simulink model "obstacle_detection"  (R2022b)
settings: Solver=VariableStepAuto  StartTime=0.0  StopTime=10.0  RelTol=1e-3
values from neighbouring files (symbols this model uses):
  m = 12    [mpc.m]    (also in mpc_soln.m; qp_soln.m)
  N = 50    [mpc.m]    (also in mpc_caller.m = 20; qp_caller.m = params.N)
  X = [p; reshape(R, [9 1]); v; R'*w]    [mpc_caller.m]    (also in qp_caller.m)
undefined symbols (not defined in the file or in its folder): Y, Z
libraries: sm_lib x269, nesl_utility x117, simulink x2
(part 5 of 5)

== system obstacle_detection/q_dot ==
  RR_calf : Inport
  RL_calf : Inport  Port=2
  FR_calf : Inport  Port=3
  FL_calf : Inport  Port=4
  RR_thigh : Inport  Port=5
  RL_thigh : Inport  Port=6
  FR_thigh : Inport  Port=7
  FL_thigh : Inport  Port=8
  RR_hip : Inport  Port=9
  RL_hip : Inport  Port=10
  FR_hip : Inport  Port=11
  FL_hip : Inport  Port=12
  Scope : Scope  NumInputPorts=12
  Vector Concatenate : Concatenate  NumInputs=12
  joint vector : Outport
  wires:
  Vector Concatenate/1 -> joint vector/1
  FR_thigh/1 -> Scope/7, Vector Concatenate/7
  FL_hip/1 -> Scope/12, Vector Concatenate/12
  FL_calf/1 -> Scope/4, Vector Concatenate/4
  FL_thigh/1 -> Scope/8, Vector Concatenate/8
  FR_hip/1 -> Scope/11, Vector Concatenate/11
  RR_calf/1 -> Scope/1, Vector Concatenate/1
  RL_hip/1 -> Scope/10, Vector Concatenate/10
  FR_calf/1 -> Scope/3, Vector Concatenate/3
  RR_thigh/1 -> Scope/5, Vector Concatenate/5
  RL_calf/1 -> Scope/2, Vector Concatenate/2
  RL_thigh/1 -> Scope/6, Vector Concatenate/6
  RR_hip/1 -> Scope/9, Vector Concatenate/9

== system obstacle_detection/qd ==
  RR_calf : Inport
  RL_calf : Inport  Port=2
  FR_calf : Inport  Port=3
  FL_calf : Inport  Port=4
  RR_thigh : Inport  Port=5
  RL_thigh : Inport  Port=6
  FR_thigh : Inport  Port=7
  FL_thigh : Inport  Port=8
  RR_hip : Inport  Port=9
  RL_hip : Inport  Port=10
  FR_hip : Inport  Port=11
  FL_hip : Inport  Port=12
  Vector Concatenate : Concatenate  NumInputs=12
  Joint vector : Outport
  wires:
  Vector Concatenate/1 -> Joint vector/1
  FR_hip/1 -> Vector Concatenate/11
  RL_calf/1 -> Vector Concatenate/2
  FL_calf/1 -> Vector Concatenate/4
  RL_thigh/1 -> Vector Concatenate/6
  FL_thigh/1 -> Vector Concatenate/8
  RR_calf/1 -> Vector Concatenate/1
  RR_hip/1 -> Vector Concatenate/9
  FR_calf/1 -> Vector Concatenate/3
  RR_thigh/1 -> Vector Concatenate/5
  FL_hip/1 -> Vector Concatenate/12
  RL_hip/1 -> Vector Concatenate/10
  FR_thigh/1 -> Vector Concatenate/7

== system obstacle_detection/tau ==
  RR_calf : Inport
  RL_calf : Inport  Port=2
  FR_calf : Inport  Port=3
  FL_calf : Inport  Port=4
  RR_thigh : Inport  Port=5
  RL_thigh : Inport  Port=6
  FR_thigh : Inport  Port=7
  FL_thigh : Inport  Port=8
  RR_hip : Inport  Port=9
  RL_hip : Inport  Port=10
  FR_hip : Inport  Port=11
  FL_hip : Inport  Port=12
  Joint Torques : Scope  NumInputPorts=12
  Vector Concatenate : Concatenate  NumInputs=12
  joint vector : Outport
  wires:
  Vector Concatenate/1 -> joint vector/1
  FR_thigh/1 -> Joint Torques/7, Vector Concatenate/7
  FL_hip/1 -> Joint Torques/12, Vector Concatenate/12
  FL_calf/1 -> Joint Torques/4, Vector Concatenate/4
  FL_thigh/1 -> Joint Torques/8, Vector Concatenate/8
  FR_hip/1 -> Joint Torques/11, Vector Concatenate/11
  RR_calf/1 -> Joint Torques/1, Vector Concatenate/1
  RL_hip/1 -> Joint Torques/10, Vector Concatenate/10
  FR_calf/1 -> Joint Torques/3, Vector Concatenate/3
  RR_thigh/1 -> Joint Torques/5, Vector Concatenate/5
  RL_calf/1 -> Joint Torques/2, Vector Concatenate/2
  RL_thigh/1 -> Joint Torques/6, Vector Concatenate/6
  RR_hip/1 -> Joint Torques/9, Vector Concatenate/9

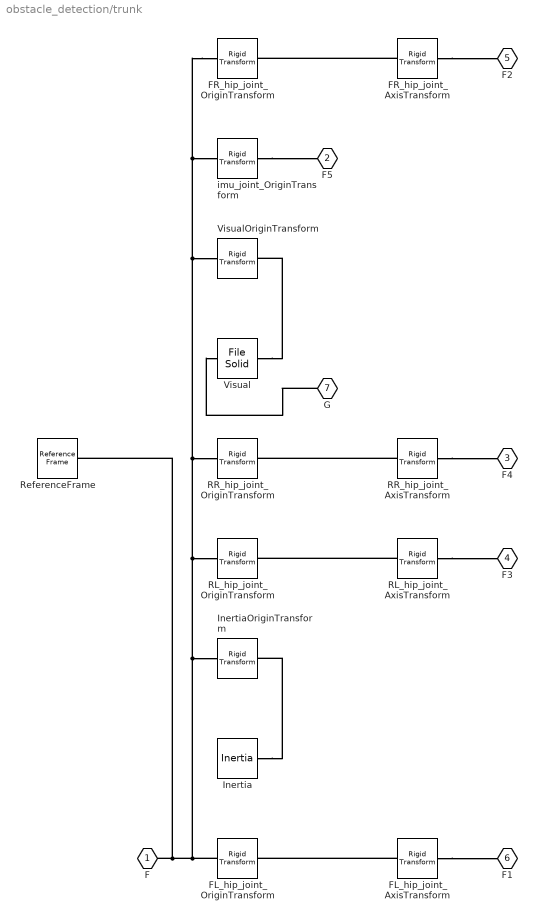
== system obstacle_detection/trunk ==
  FL_hip_joint_AxisTransform : sm_lib/Frames and Transforms/Rigid Transform  TranslationMethod=Cartesian  TranslationStandardOffset=0  TranslationLengthUnit=m  TranslationStandardAxis=+Z  TranslationCartesianOffset=[0, 0, 0]  TranslationROffset=0  TranslationROffsetUnits=m  TranslationZOffset=0  TranslationZOffsetUnits=m  TranslationThetaOffset=0  TranslationThetaOffsetUnits=deg  RotationMethod=ArbitraryAxis  RotationAngleUnits=rad  RotationStandardAxis=+Z  RotationAngle=1.570796326794897  RotationArbitraryAxis=[-0, 1, 0]  FollAlignAxisA=+X  BaseAlignAxisA=+Y  FollAlignAxisB=+Y  BaseAlignAxisB=+Z  RotationSequenceAxes=FollowerAxes  RotationSequence=XYX  RotationSequenceAngles=[0 0 0]  RotationSequenceAnglesUnits=deg  RotationMatrix=[1 0 0; 0 1 0; 0 0 1]  Quaternion=[1 0 0 0]
  FL_hip_joint_OriginTransform : sm_lib/Frames and Transforms/Rigid Transform  TranslationMethod=Cartesian  TranslationStandardOffset=0  TranslationLengthUnit=m  TranslationStandardAxis=+Z  TranslationCartesianOffset=[0.1805, 0.047, 0]  TranslationROffset=0  TranslationROffsetUnits=m  TranslationZOffset=0  TranslationZOffsetUnits=m  TranslationThetaOffset=0  TranslationThetaOffsetUnits=deg  RotationMethod=RotationSequence  RotationAngleUnits=deg  RotationStandardAxis=+Z  RotationAngle=0.0  RotationArbitraryAxis=[0 0 1]  FollAlignAxisA=+X  BaseAlignAxisA=+Y  FollAlignAxisB=+Y  BaseAlignAxisB=+Z  RotationSequenceAxes=BaseAxes  RotationSequence=XYZ  RotationSequenceAngles=[0, 0, 0]  RotationSequenceAnglesUnits=rad  RotationMatrix=[1 0 0; 0 1 0; 0 0 1]  Quaternion=[1 0 0 0]
  FR_hip_joint_AxisTransform : sm_lib/Frames and Transforms/Rigid Transform  TranslationMethod=Cartesian  TranslationStandardOffset=0  TranslationLengthUnit=m  TranslationStandardAxis=+Z  TranslationCartesianOffset=[0, 0, 0]  TranslationROffset=0  TranslationROffsetUnits=m  TranslationZOffset=0  TranslationZOffsetUnits=m  TranslationThetaOffset=0  TranslationThetaOffsetUnits=deg  RotationMethod=ArbitraryAxis  RotationAngleUnits=rad  RotationStandardAxis=+Z  RotationAngle=1.570796326794897  RotationArbitraryAxis=[-0, 1, 0]  FollAlignAxisA=+X  BaseAlignAxisA=+Y  FollAlignAxisB=+Y  BaseAlignAxisB=+Z  RotationSequenceAxes=FollowerAxes  RotationSequence=XYX  RotationSequenceAngles=[0 0 0]  RotationSequenceAnglesUnits=deg  RotationMatrix=[1 0 0; 0 1 0; 0 0 1]  Quaternion=[1 0 0 0]
  FR_hip_joint_OriginTransform : sm_lib/Frames and Transforms/Rigid Transform  TranslationMethod=Cartesian  TranslationStandardOffset=0  TranslationLengthUnit=m  TranslationStandardAxis=+Z  TranslationCartesianOffset=[0.1805, -0.047, 0]  TranslationROffset=0  TranslationROffsetUnits=m  TranslationZOffset=0  TranslationZOffsetUnits=m  TranslationThetaOffset=0  TranslationThetaOffsetUnits=deg  RotationMethod=RotationSequence  RotationAngleUnits=deg  RotationStandardAxis=+Z  RotationAngle=0.0  RotationArbitraryAxis=[0 0 1]  FollAlignAxisA=+X  BaseAlignAxisA=+Y  FollAlignAxisB=+Y  BaseAlignAxisB=+Z  RotationSequenceAxes=BaseAxes  RotationSequence=XYZ  RotationSequenceAngles=[0, 0, 0]  RotationSequenceAnglesUnits=rad  RotationMatrix=[1 0 0; 0 1 0; 0 0 1]  Quaternion=[1 0 0 0]
  Inertia : sm_lib/Body Elements/Inertia  InertiaType=Custom  Mass=6  MassUnits=kg  CenterOfMass=[0, 0, 0]  CenterOfMassUnits=m  MomentsOfInertia=[0.0158533, 0.0377999, 0.0456542]  MomentsOfInertiaUnits=kg*m^2  ProductsOfInertia=[-2.75e-05, -6.109999999999999e-05, -3.66e-05]  ProductsOfInertiaUnits=kg*m^2  GraphicType=None  MarkerShape=Inertia  MarkerSize=20  GraphicVisPropType=SimpleVisualProperties  GraphicDiffuseColor=[0.5 0.5 0.5]  GraphicSpecularColor=[0.5 0.5 0.5 1.0]  GraphicAmbientColor=[0.15 0.15 0.15 1.0]  GraphicEmissiveColor=[0.0 0.0 0.0 1.0]  GraphicShininess=75  GraphicOpacity=1.0
  InertiaOriginTransform : sm_lib/Frames and Transforms/Rigid Transform  TranslationMethod=Cartesian  TranslationStandardOffset=0  TranslationLengthUnit=m  TranslationStandardAxis=+Z  TranslationCartesianOffset=[0, 0.0041, -0.0005]  TranslationROffset=0  TranslationROffsetUnits=m  TranslationZOffset=0  TranslationZOffsetUnits=m  TranslationThetaOffset=0  TranslationThetaOffsetUnits=deg  RotationMethod=RotationSequence  RotationAngleUnits=deg  RotationStandardAxis=+Z  RotationAngle=0.0  RotationArbitraryAxis=[0 0 1]  FollAlignAxisA=+X  BaseAlignAxisA=+Y  FollAlignAxisB=+Y  BaseAlignAxisB=+Z  RotationSequenceAxes=BaseAxes  RotationSequence=XYZ  RotationSequenceAngles=[0, 0, 0]  RotationSequenceAnglesUnits=rad  RotationMatrix=[1 0 0; 0 1 0; 0 0 1]  Quaternion=[1 0 0 0]
  RL_hip_joint_AxisTransform : sm_lib/Frames and Transforms/Rigid Transform  TranslationMethod=Cartesian  TranslationStandardOffset=0  TranslationLengthUnit=m  TranslationStandardAxis=+Z  TranslationCartesianOffset=[0, 0, 0]  TranslationROffset=0  TranslationROffsetUnits=m  TranslationZOffset=0  TranslationZOffsetUnits=m  TranslationThetaOffset=0  TranslationThetaOffsetUnits=deg  RotationMethod=ArbitraryAxis  RotationAngleUnits=rad  RotationStandardAxis=+Z  RotationAngle=1.570796326794897  RotationArbitraryAxis=[-0, 1, 0]  FollAlignAxisA=+X  BaseAlignAxisA=+Y  FollAlignAxisB=+Y  BaseAlignAxisB=+Z  RotationSequenceAxes=FollowerAxes  RotationSequence=XYX  RotationSequenceAngles=[0 0 0]  RotationSequenceAnglesUnits=deg  RotationMatrix=[1 0 0; 0 1 0; 0 0 1]  Quaternion=[1 0 0 0]
  RL_hip_joint_OriginTransform : sm_lib/Frames and Transforms/Rigid Transform  TranslationMethod=Cartesian  TranslationStandardOffset=0  TranslationLengthUnit=m  TranslationStandardAxis=+Z  TranslationCartesianOffset=[-0.1805, 0.047, 0]  TranslationROffset=0  TranslationROffsetUnits=m  TranslationZOffset=0  TranslationZOffsetUnits=m  TranslationThetaOffset=0  TranslationThetaOffsetUnits=deg  RotationMethod=RotationSequence  RotationAngleUnits=deg  RotationStandardAxis=+Z  RotationAngle=0.0  RotationArbitraryAxis=[0 0 1]  FollAlignAxisA=+X  BaseAlignAxisA=+Y  FollAlignAxisB=+Y  BaseAlignAxisB=+Z  RotationSequenceAxes=BaseAxes  RotationSequence=XYZ  RotationSequenceAngles=[0, 0, 0]  RotationSequenceAnglesUnits=rad  RotationMatrix=[1 0 0; 0 1 0; 0 0 1]  Quaternion=[1 0 0 0]
  RR_hip_joint_AxisTransform : sm_lib/Frames and Transforms/Rigid Transform  TranslationMethod=Cartesian  TranslationStandardOffset=0  TranslationLengthUnit=m  TranslationStandardAxis=+Z  TranslationCartesianOffset=[0, 0, 0]  TranslationROffset=0  TranslationROffsetUnits=m  TranslationZOffset=0  TranslationZOffsetUnits=m  TranslationThetaOffset=0  TranslationThetaOffsetUnits=deg  RotationMethod=ArbitraryAxis  RotationAngleUnits=rad  RotationStandardAxis=+Z  RotationAngle=1.570796326794897  RotationArbitraryAxis=[-0, 1, 0]  FollAlignAxisA=+X  BaseAlignAxisA=+Y  FollAlignAxisB=+Y  BaseAlignAxisB=+Z  RotationSequenceAxes=FollowerAxes  RotationSequence=XYX  RotationSequenceAngles=[0 0 0]  RotationSequenceAnglesUnits=deg  RotationMatrix=[1 0 0; 0 1 0; 0 0 1]  Quaternion=[1 0 0 0]
  RR_hip_joint_OriginTransform : sm_lib/Frames and Transforms/Rigid Transform  TranslationMethod=Cartesian  TranslationStandardOffset=0  TranslationLengthUnit=m  TranslationStandardAxis=+Z  TranslationCartesianOffset=[-0.1805, -0.047, 0]  TranslationROffset=0  TranslationROffsetUnits=m  TranslationZOffset=0  TranslationZOffsetUnits=m  TranslationThetaOffset=0  TranslationThetaOffsetUnits=deg  RotationMethod=RotationSequence  RotationAngleUnits=deg  RotationStandardAxis=+Z  RotationAngle=0.0  RotationArbitraryAxis=[0 0 1]  FollAlignAxisA=+X  BaseAlignAxisA=+Y  FollAlignAxisB=+Y  BaseAlignAxisB=+Z  RotationSequenceAxes=BaseAxes  RotationSequence=XYZ  RotationSequenceAngles=[0, 0, 0]  RotationSequenceAnglesUnits=rad  RotationMatrix=[1 0 0; 0 1 0; 0 0 1]  Quaternion=[1 0 0 0]
  ReferenceFrame : sm_lib/Frames and Transforms/Reference Frame
  Visual : sm_lib/Body Elements/File Solid  ExtGeomFileName=meshes/trunk.stl  UnitType=Custom  ExtGeomFileUnits=m  StepReaderType=HEX  ExportConvexHullGeometry=on  InertiaType=Custom  Mass=0  MassUnits=kg  CenterOfMass=[0, 0, 0]  CenterOfMassUnits=m  MomentsOfInertia=[0, 0, 0]  MomentsOfInertiaUnits=kg*m^2  ProductsOfInertia=[0, 0, 0]  ProductsOfInertiaUnits=kg*m^2  BasedOnType=DensityFromFile  Density=1000  DensityUnits=kg/m^3  DoExposeReferenceFrame=on  SerializedFrames=<Frames/>  GraphicType=FromGeometry  MarkerShape=Sphere  MarkerSize=10  GraphicVisPropType=SimpleVisualProperties  GraphicDiffuseColor=[0.8 1.0 1.0]  GraphicSpecularColor=[0.5 0.5 0.5 1.0]  GraphicAmbientColor=[0.15 0.15 0.15 1.0]  GraphicEmissiveColor=[0.0 0.0 0.0 1.0]  GraphicShininess=75  GraphicOpacity=1
  VisualOriginTransform : sm_lib/Frames and Transforms/Rigid Transform  TranslationMethod=Cartesian  TranslationStandardOffset=0  TranslationLengthUnit=m  TranslationStandardAxis=+Z  TranslationCartesianOffset=[0, 0, 0]  TranslationROffset=0  TranslationROffsetUnits=m  TranslationZOffset=0  TranslationZOffsetUnits=m  TranslationThetaOffset=0  TranslationThetaOffsetUnits=deg  RotationMethod=RotationSequence  RotationAngleUnits=deg  RotationStandardAxis=+Z  RotationAngle=0.0  RotationArbitraryAxis=[0 0 1]  FollAlignAxisA=+X  BaseAlignAxisA=+Y  FollAlignAxisB=+Y  BaseAlignAxisB=+Z  RotationSequenceAxes=BaseAxes  RotationSequence=XYZ  RotationSequenceAngles=[0, 0, 0]  RotationSequenceAnglesUnits=rad  RotationMatrix=[1 0 0; 0 1 0; 0 0 1]  Quaternion=[1 0 0 0]
  imu_joint_OriginTransform : sm_lib/Frames and Transforms/Rigid Transform  TranslationMethod=Cartesian  TranslationStandardOffset=0  TranslationLengthUnit=m  TranslationStandardAxis=+Z  TranslationCartesianOffset=[0, 0, 0]  TranslationROffset=0  TranslationROffsetUnits=m  TranslationZOffset=0  TranslationZOffsetUnits=m  TranslationThetaOffset=0  TranslationThetaOffsetUnits=deg  RotationMethod=RotationSequence  RotationAngleUnits=deg  RotationStandardAxis=+Z  RotationAngle=0.0  RotationArbitraryAxis=[0 0 1]  FollAlignAxisA=+X  BaseAlignAxisA=+Y  FollAlignAxisB=+Y  BaseAlignAxisB=+Z  RotationSequenceAxes=BaseAxes  RotationSequence=XYZ  RotationSequenceAngles=[0, 0, 0]  RotationSequenceAnglesUnits=rad  RotationMatrix=[1 0 0; 0 1 0; 0 0 1]  Quaternion=[1 0 0 0]
  F : PMIOPort  Side=Left
  F5 : PMIOPort  Port=2  Side=Right
  F4 : PMIOPort  Port=3  Side=Right
  F3 : PMIOPort  Port=4  Side=Right
  F2 : PMIOPort  Port=5  Side=Right
  F1 : PMIOPort  Port=6  Side=Right
  G : PMIOPort  Port=7  Side=Right
  connections:
  FL_hip_joint_AxisTransform/RConn1 -- F1/RConn1
  FL_hip_joint_AxisTransform/LConn1 -- FL_hip_joint_OriginTransform/RConn1
  FR_hip_joint_AxisTransform/RConn1 -- F2/RConn1
  FR_hip_joint_AxisTransform/LConn1 -- FR_hip_joint_OriginTransform/RConn1
  Inertia/RConn1 -- InertiaOriginTransform/RConn1
  RL_hip_joint_AxisTransform/RConn1 -- F3/RConn1
  RL_hip_joint_AxisTransform/LConn1 -- RL_hip_joint_OriginTransform/RConn1
  RR_hip_joint_AxisTransform/RConn1 -- F4/RConn1
  RR_hip_joint_AxisTransform/LConn1 -- RR_hip_joint_OriginTransform/RConn1
  FR_hip_joint_OriginTransform/LConn1 -- FL_hip_joint_OriginTransform/LConn1 -- ReferenceFrame/RConn1 -- F/RConn1 -- InertiaOriginTransform/LConn1 -- RL_hip_joint_OriginTransform/LConn1 -- RR_hip_joint_OriginTransform/LConn1 -- VisualOriginTransform/LConn1 -- imu_joint_OriginTransform/LConn1
  Visual/RConn1 -- VisualOriginTransform/RConn1
  imu_joint_OriginTransform/RConn1 -- F5/RConn1
  G/RConn1 -- Visual/LConn1

== system obstacle_detection/vd_COM ==
  Constant3 : Constant  Value=0
  Ramp : simulink/Sources/Ramp  slope=0.2  start=1.95  InitialOutput=0.2
  Saturation1 : Saturate  UpperLimit=0.2  LowerLimit=-0.6
  Vector Concatenate3 : Concatenate  NumInputs=3
  Out1 : Outport
  wires:
  Constant3/1 -> Vector Concatenate3/2, Vector Concatenate3/3
  Saturation1/1 -> Vector Concatenate3/1
  Vector Concatenate3/1 -> Out1/1
  Ramp/1 -> Saturation1/1

== matlab function obstacle_detection/Subsystem13/MATLAB Function1 ==
  data: p input; v input; w input; tau output; R input; q input; vd input; p1 input; p2 input; p3 input; p4 input; t input; F output; task input; z output
function [tau, F, z] = mpc_controller_wrapper(p, v, w, R, q, vd, p1, p2, p3, p4, t, task)
    [tau, F, z] = mpc_caller(p, v, w, R, q, vd, p1, p2, p3, p4, t, task);
end

== matlab function obstacle_detection/MATLAB Function ==
  data: q input; tau output; q_dot input; qd input; qd_dot input
function tau = pd_controller(q, q_dot, qd, qd_dot)
    Kp = 1e3; Kd = 1e3;
    
    tau = Kp * (qd - q) + Kd * (qd_dot - q_dot);

== matlab function obstacle_detection/MATLAB Function1 ==
  data: tau_pd input; tau output; tau_mpc input; tau_swing input; tau_qp input; q input; q_dot input; qd input; qd_dot input; t input
function tau = choose_controller(tau_pd, tau_mpc, tau_swing, tau_qp, q, q_dot, qd, qd_dot, t)

select_leg = [0;0;1;0];

if t >= get_gait_params().t_start
    tau = tau_mpc + tau_swing;
%     tau = tau_mpc + tau_swing.*[select_leg;select_leg;select_leg;];
    %tau = tau_pd.*[1-select_leg; 1-select_leg; 1-select_leg] + tau_swing.*[select_leg; select_leg; select_leg];
    %tau = tau_qp.*[1-select_leg; 1-select_leg; 1-select_leg] + tau_swing.*[select_leg; select_leg; select_leg];

else
    tau = tau_qp;
end

== matlab function obstacle_detection/MATLAB Function2 ==
  data: p input; R input; tau output; v input; p_hip input; p_foot_initial input; p_foot input; v_foot input; q input; vd input; w input; t input; pd_foot output; vd_foot output; pfinal_foot output; Fswing output; task input
function [tau, pd_foot, vd_foot, pfinal_foot, Fswing]   = swing_controller(p, R, v, p_hip, p_foot_initial, p_foot, v_foot, q, vd, w, t, task)

tau = zeros(12,1);
pd_foot = zeros(12,1);
vd_foot = zeros(12,1);
Fswing = zeros(12,1);
pfinal_foot = zeros(12,1);

if task == 0 % standing
    [tau, pd_foot, vd_foot, Fswing] = foot_placement_standing(p, R, v, p_hip, p_foot, v_foot, q, t);
elseif task == 1 % walking
    [tau, pd_foot, vd_foot, pfinal_foot, Fswing] = foot_placement_walking(p, R, v, p_hip, p_foot, v_foot, q, vd, t);
elseif task == 2 % turning
    [tau, pd_foot, vd_foot, pfinal_foot, Fswing] = foot_placement_turning(p, R, v, p_hip, p_foot, v_foot, q, vd, t);
elseif task == 5 % climbing
    [tau, pd_foot, vd_foot, pfinal_foot, Fswing] = foot_placement_climbing(p, R, v, p_hip, p_foot_initial, p_foot, v_foot, q, vd, t);
end


% select_leg = [0;0;1;0];
% tau = tau.*[select_leg;select_leg;select_leg;]

== matlab function obstacle_detection/MATLAB Function3 ==
  data: p input; v input; w input; tau output; R input; q input; p1 input; p2 input; p3 input; p4 input; t input; F output
function [tau, F] = qp_controller_wrapper(p, v, w, R, q, p1, p2, p3, p4, t)
    [tau, F] = qp_caller(p, v, w, R, q, p1, p2, p3, p4, t);
end
